simulink library "Vessel"  (R2023a)
settings: Solver=VariableStepAuto  StartTime=0.0  StopTime=10.0  RelTol=1e-3
undefined symbols (not defined in the file): A_ann_aor, alpha1, alpha2, atrium_ventricle, BSA, control, conversion_factor, DAP, DLVP, DP_close_aor, DP_open_aor, DPP, DRVP, E0, E_max, E_min, E_sa_0, E_sv_0, eta, g, K_vc_aor, K_vo_aor, l, L0, lambda, m1, m2, M_rg_aor, M_st_aor, MAP, MPP, n, P0, p_septum_on_off, p_th_on_off, phi, PVR, Q_max, rho, SAP, SI, sigma, SLVP, SPP, SRVP, SVR, t_delay, Ts, UVV_0, V0, V_0, V_max, V_tot, Y_aorta, Y_control
libraries: $bdroot x100, simulink x39, dspsigops x20, slpidlib x11, eeGeneralControl x2, dspstat3 x1
(part 4 of 4)

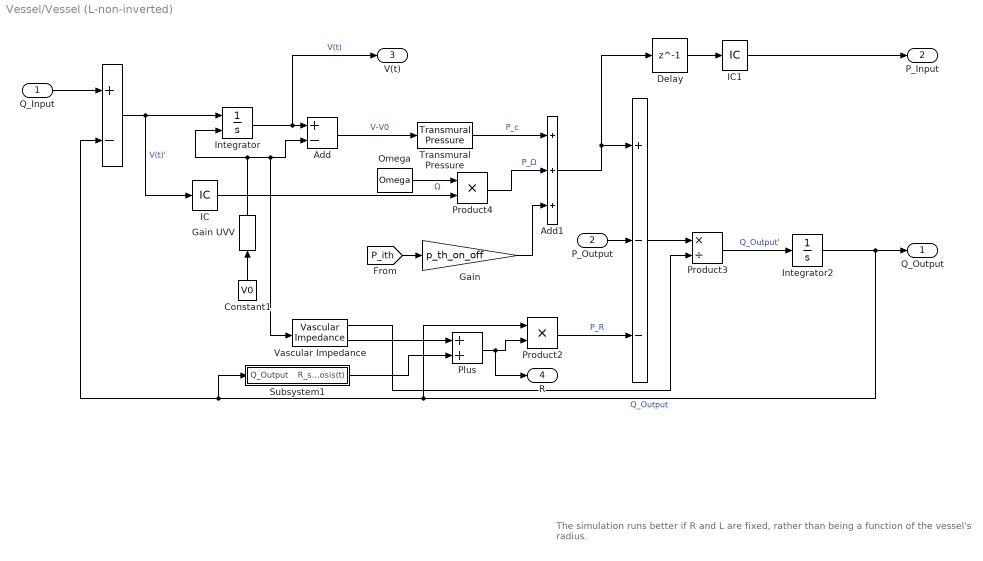
== system Vessel/Vessel (L-non-inverted)  ==
  note: The simulation runs better if R and L are fixed, rather than being a function of the vessel's radius.
  Q_Input : Inport
  P_Output : Inport  Port=2  Unit=mmHg
  " " : Sum  Inputs=+--
  "   " : Sum  Inputs=+-
  Add : Sum  Inputs=+-
  Add1 : Sum  Inputs=+++
  Constant1 : Constant  Value=V0
  Delay : Delay  DelayLength=1  InitialCondition=P0
  Gain : Gain  Gain=p_th_on_off
  Gain UVV : $bdroot/Gain UVV  SystemSampleTime=-1  VariantActivationTime=update diagram  Latency=0  AutoFrameSizeCalculation=off
  IC : InitialCondition  Value=0
  IC1 : InitialCondition  Value=P0
  Integrator : Integrator  InitialConditionSource=external  LimitOutput=on  LowerSaturationLimit=0  ContinuousStateAttributes='Volume'
  Integrator2 : Integrator  LimitOutput=on  UpperSaturationLimit=4000  LowerSaturationLimit=-4000  ContinuousStateAttributes='Flow'
  Omega : $bdroot/Omega  SystemSampleTime=-1  VariantActivationTime=update diagram  Latency=0  AutoFrameSizeCalculation=off
  Plus : Sum
  Product2 : Product
  Product3 : Product  Inputs=*/
  Product4 : Product
  Subsystem1 : Subsystem
  Transmural Pressure : $bdroot/Transmural Pressure  SystemSampleTime=-1  VariantActivationTime=update diagram  Latency=0  AutoFrameSizeCalculation=off
  Vascular Impedance : $bdroot/Vascular Impedance  SystemSampleTime=-1  VariantActivationTime=update diagram  Latency=0  AutoFrameSizeCalculation=off
  Q_Output : Outport
  P_Input : Outport  Port=2
  V(t) : Outport  Port=3
  R : Outport  Port=4
  wires:
  Constant1/1 -> Gain UVV/1
  Integrator2/1 -> Q_Output/1, Product2/1, Subsystem1/1(Q_Output), "   "/2  "Q_Output"
  P_Output/1 -> " "/2
  Omega/1 -> Product4/1  "Ω"
  Product4/1 -> Add1/2  "P_Ω"
  Q_Input/1 -> "   "/1
  Transmural Pressure/1 -> Add1/1  "P_c"
  Add1/1 -> Delay/1, " "/1
  " "/1 -> Product3/1
  Product2/1 -> " "/3  "P_R"
  Add/1 -> Transmural Pressure/1  "V-V0"
  Integrator/1 -> V(t)/1, Add/1  "V(t)"
  "   "/1 -> IC/1, Integrator/1  "V(t)'"
  Product3/1 -> Integrator2/1  "Q_Output'"
  Vascular Impedance/1 -> Product3/2
  [P_ith] -> Gain/1
  Gain/1 -> Add1/3
  IC/1 -> Product4/2
  IC1/1 -> P_Input/1
  Delay/1 -> IC1/1
  Vascular Impedance/2 -> Plus/1
  Plus/1 -> R/1, Product2/2
  Subsystem1/1(R_stenosis(t)) -> Plus/2
  Gain UVV/1 -> Integrator/2, Vascular Impedance/1, Add/2

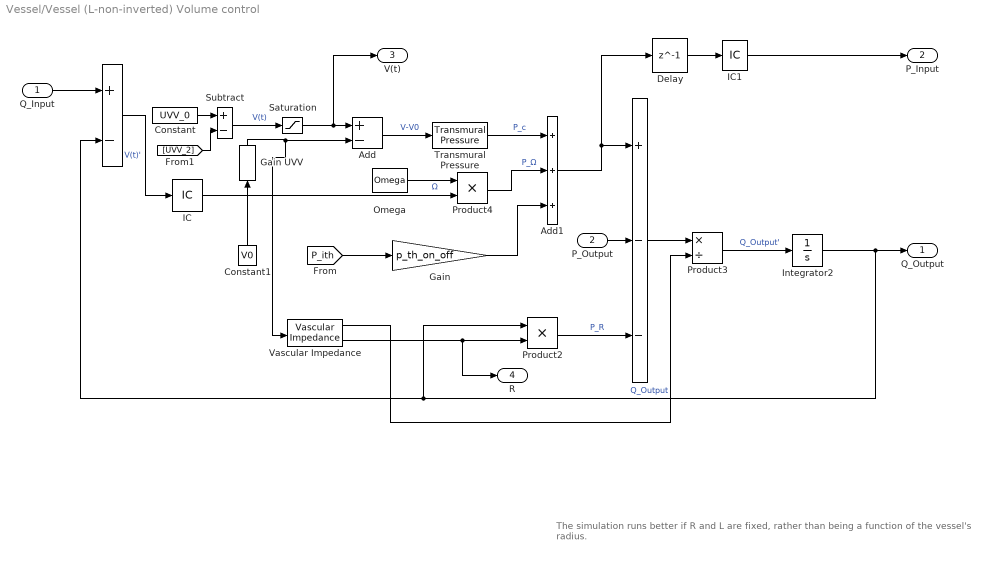
== system Vessel/Vessel (L-non-inverted) Volume control ==
  note: The simulation runs better if R and L are fixed, rather than being a function of the vessel's radius.
  Q_Input : Inport
  P_Output : Inport  Port=2  Unit=mmHg
  " " : Sum  Inputs=+--
  "   " : Sum  Inputs=+-
  Add : Sum  Inputs=+-
  Add1 : Sum  Inputs=+++
  Constant : Constant  Value=UVV_0
  Constant1 : Constant  Value=V0
  Delay : Delay  DelayLength=1  InitialCondition=P0
  Gain : Gain  Gain=p_th_on_off
  Gain UVV : $bdroot/Gain UVV  SystemSampleTime=-1  VariantActivationTime=update diagram  Latency=0  AutoFrameSizeCalculation=off
  IC : InitialCondition  Value=0
  IC1 : InitialCondition  Value=P0
  Integrator2 : Integrator  LimitOutput=on  UpperSaturationLimit=4000  LowerSaturationLimit=-4000  ContinuousStateAttributes='Flow'
  Omega : $bdroot/Omega  SystemSampleTime=-1  VariantActivationTime=update diagram  Latency=0  AutoFrameSizeCalculation=off
  Product2 : Product
  Product3 : Product  Inputs=*/
  Product4 : Product
  Saturation : Saturate  UpperLimit=inf  LowerLimit=0
  Subtract : Sum  Inputs=+-
  Transmural Pressure : $bdroot/Transmural Pressure  SystemSampleTime=-1  VariantActivationTime=update diagram  Latency=0  AutoFrameSizeCalculation=off
  Vascular Impedance : $bdroot/Vascular Impedance  SystemSampleTime=-1  VariantActivationTime=update diagram  Latency=0  AutoFrameSizeCalculation=off
  Q_Output : Outport
  P_Input : Outport  Port=2
  V(t) : Outport  Port=3
  R : Outport  Port=4
  wires:
  Delay/1 -> IC1/1
  IC1/1 -> P_Input/1
  Gain/1 -> Add1/3
  [P_ith] -> Gain/1
  Vascular Impedance/1 -> Product3/2
  Vascular Impedance/2 -> R/1, Product2/2
  Product3/1 -> Integrator2/1  "Q_Output'"
  "   "/1 -> IC/1  "V(t)'"
  Subtract/1 -> Saturation/1  "V(t)"
  Add/1 -> Transmural Pressure/1  "V-V0"
  Product2/1 -> " "/3  "P_R"
  " "/1 -> Product3/1
  Add1/1 -> " "/1, Delay/1
  Transmural Pressure/1 -> Add1/1  "P_c"
  Q_Input/1 -> "   "/1
  Product4/1 -> Add1/2  "P_Ω"
  Omega/1 -> Product4/1  "Ω"
  P_Output/1 -> " "/2
  Integrator2/1 -> "   "/2, Product2/1, Q_Output/1  "Q_Output"
  Constant1/1 -> Gain UVV/1
  [UVV_2] -> Subtract/2
  Constant/1 -> Subtract/1
  Saturation/1 -> Add/1, V(t)/1
  IC/1 -> Product4/2
  Gain UVV/1 -> Vascular Impedance/1, Add/2

== system Vessel/Volume Control ==
  note: OLD
  V_tot(t) : Inport
  Add : Sum  Commented=on
  Constant : Constant  Value=V_tot_0
  Filtered Derivative (Discrete or Continuous) : eeGeneralControl/Filtered Derivative (Discrete or Continuous)  Commented=on  K=1  T=Ts  B=inf  A=-inf  minRatio=1  init_option=Inherited from block input  x0=0  Ts=-1
      settings: LibrarySourceBlock=|
      | ee_sl_lib/General Control/Filtered Derivative
      | (Discrete or Continuous)
  Moving Average : dspstat3/Moving Average  Commented=on  Method=Sliding window  ForgettingFactorPort=off  SpecifyWindowLength=on  WindowLength=4  OverlapLength=3  AllowArbitraryInputLength=off  ForgettingFactor=0.9  SimulateUsing=Code generation
  Subtract : Sum  Inputs=+-
  Switch1 : Switch  Criteria=u2 > Threshold  SaturateOnIntegerOverflow=off  InputSameDT=off
  Q_output : Outport
  wires:
  [V_tot] -> Subtract/2
  Switch1/1 -> Subtract/1
  Subtract/1 -> Q_output/1  "V(t)"
  Filtered Derivative (Discrete or Continuous)/1 -> Add/1
  Constant/1 -> Switch1/3
  V_tot(t)/1 -> Switch1/2, Switch1/1
  Moving Average/1 -> Add/2

== system Vessel/Baroflex control (Fresiello)/Afferent sympathetic activity ==
  P(t) : Inport
  Constant1 : Constant  Value=A*WL
  Constant2 : Constant
  Constant3 : Constant  Value=Paa_SET0
  Constant4 : Constant  Value=Fas_min
  Divide : Product  Inputs=*/
  Gain : Gain  Gain=1/ka
  Gain1 : Gain  Gain=Fas_max
  Math Function : Math
  Minus : Sum  Inputs=-+
  Minus1 : Sum
  Minus2 : Sum
  Minus3 : Sum
  Fas(t) : Outport
  wires:
  Minus1/1 -> Divide/1
  Divide/1 -> Fas(t)/1
  Constant2/1 -> Minus2/2
  Constant4/1 -> Minus1/2
  Gain/1 -> Math Function/1
  P(t)/1 -> Minus/2
  Constant3/1 -> Minus3/2
  Minus/1 -> Gain/1
  Math Function/1 -> Gain1/1, Minus2/1
  Gain1/1 -> Minus1/1
  Minus2/1 -> Divide/2
  Constant1/1 -> Minus3/1
  Minus3/1 -> Minus/1  "Paa_SET"

== system Vessel/Baroflex control (Fresiello)/Efferent sympathetic nerve activity ==
  Fas(t) : Inport
  Constant1 : Constant  Value=B*WL
  Constant4 : Constant  Value=Fes_inf
  Gain : Gain  Gain=-kes
  Gain1 : Gain  Gain=Fes_0-Fes_inf
  Math Function : Math
  Minus2 : Sum  Inputs=+++
  " Fes(t)" : Outport
  wires:
  Math Function/1 -> Gain1/1
  Gain/1 -> Math Function/1
  Fas(t)/1 -> Gain/1
  Gain1/1 -> Minus2/1
  Constant4/1 -> Minus2/2
  Constant1/1 -> Minus2/3  "Δ_Fes"
  Minus2/1 -> " Fes(t)"/1

== system Vessel/Baroflex control (Fresiello)/Efferent vagal nerve activity ==
  Fas(t) : Inport
  " " : Product  Inputs=**
  Constant : Constant
  Constant1 : Constant  Value=C*WL
  Constant2 : Constant  Value=Fas_0
  Constant3 : Constant  Value=Fev_inf0+D*WL
  Constant4 : Constant  Value=Fev_0
  Divide : Product  Inputs=*/
  Gain : Gain  Gain=1/kev
  Math Function : Math
  Minus1 : Sum  Inputs=+-
  Minus2 : Sum
  Minus3 : Sum
  Minus4 : Sum
  " Fev(t)" : Outport
  wires:
  Minus2/1 -> Divide/1
  Constant1/1 -> Minus4/2  "Δ_Fev"
  Constant4/1 -> Minus2/2
  " "/1 -> Minus2/1
  Fas(t)/1 -> Minus1/1
  Gain/1 -> Math Function/1
  Math Function/1 -> Minus3/1, " "/2
  Constant2/1 -> Minus1/2
  Minus1/1 -> Gain/1
  Minus3/1 -> Divide/2
  Constant/1 -> Minus3/2
  Divide/1 -> Minus4/1
  Minus4/1 -> " Fev(t)"/1
  Constant3/1 -> " "/1  "Fev_inf"

== system Vessel/Baroflex control (Fresiello)/Pressure derivation ==
  Paa(t) : Inport
  Filtered Derivative : eeGeneralControl/Filtered Derivative (Discrete or Continuous)  K=1  T=inf  B=inf  A=-inf  minRatio=10  init_option=Inherited from block input  x0=0  Ts=-1
  Gain : Gain  Gain=tau_z
  Gain2 : Gain  Gain=1/tau_p
  Integrator : Integrator
  Minus2 : Sum  Inputs=++-
  P(t) : Outport
  wires:
  Integrator/1 -> Minus2/3, P(t)/1  "P(t)"
  Gain2/1 -> Integrator/1  "P(t)'"
  Paa(t)/1 -> Minus2/2, Filtered Derivative/1  "Paa(t)"
  Filtered Derivative/1 -> Gain/1  "Paa(t)'"
  Gain/1 -> Minus2/1
  Minus2/1 -> Gain2/1

== system Vessel/Baroflex control (Fresiello)/Static sympathetic function ==
  Fes(t) : Inport
  Constant1 : Constant  Value=1.65
  Constant2 : Constant  Value=1.1
  Constant3 : Constant  Value=0
  Gain : Gain  Gain=C_Hs
  Math Function : Math  Operator=log
  Minus : Sum  Inputs=--+
  Minus1 : Sum  Inputs=-+
  Subsystem : Subsystem
  Switch : Switch  Criteria=u2 > Threshold  SaturateOnIntegerOverflow=off  InputSameDT=off
  Transport Delay : TransportDelay  DelayTime=D_Hs
  sf_Hs(t) : Outport
  wires:
  Fes(t)/1 -> Transport Delay/1
  Transport Delay/1 -> Minus/3
  Constant1/1 -> Minus/2
  Constant2/1 -> Minus1/1
  Gain/1 -> sf_Hs(t)/1
  Minus1/1 -> Gain/1
  Subsystem/1(" Fes_SET") -> Minus/1
  Minus/1 -> Math Function/1, Switch/2
  Math Function/1 -> Switch/1
  Switch/1 -> Minus1/2
  Constant3/1 -> Switch/3

== system Vessel/Baroflex control (Fresiello)/Static vagal function ==
  Fev(t) : Inport
  Gain : Gain  Gain=C_Hv
  Minus : Sum  Inputs=-+
  Subsystem : Subsystem
  Transport Delay : TransportDelay  DelayTime=D_Hv
  sf_Hv(t) : Outport
  wires:
  Fev(t)/1 -> Transport Delay/1
  Minus/1 -> Gain/1
  Gain/1 -> sf_Hv(t)/1
  Transport Delay/1 -> Minus/2
  Subsystem/1(" Fev_SET") -> Minus/1

== system Vessel/Carotid Artery (L-non-inverted)/Subsystem1 ==
  Q_Output : Inport
  Abs : Abs  SaturateOnIntegerOverflow=off
  Gain1 : Gain  Gain=SI
  R_stenosis(t) : Outport
  wires:
  Abs/1 -> Gain1/1
  Gain1/1 -> R_stenosis(t)/1
  Q_Output/1 -> Abs/1

== system Vessel/Coarctation (L-non-inverted)/Subsystem ==
  Q_Output : Inport
  Abs : Abs  SaturateOnIntegerOverflow=off
  Gain1 : Gain  Gain=SI*0.000750062
  R_stenosis(t) : Outport
  wires:
  Q_Output/1 -> Abs/1
  Gain1/1 -> R_stenosis(t)/1
  Abs/1 -> Gain1/1

== system Vessel/Heart Chamber1/Pericardial pressure ==
  Vpc : Inport
  Add : Sum
  Add1 : Sum  Inputs=+-+
  Constant : Constant  Value=V_pe
  Constant14 : Constant  Value=P_pc_0
  Constant15 : Constant  Value=V_pc_0
  Constant16 : Constant  Value=phi_pc
  Exp : Math
  Gain : Gain  Gain=K_pc
  Product3 : Product  Inputs=*/
  P_pc : Outport
  wires:
  Add/1 -> P_pc/1
  Exp/1 -> Gain/1
  Constant/1 -> Add1/3
  Constant14/1 -> Add/1
  Vpc/1 -> Add1/1
  Add1/1 -> Product3/1
  Constant15/1 -> Add1/2
  Gain/1 -> Add/2
  Product3/1 -> Exp/1
  Constant16/1 -> Product3/2

== system Vessel/Intrathoracic Pressure/Breathing cycle ==
  Clock : Clock
  Constant : Constant  Value=t_exp+t_ins
  Mod : Math  Operator=mod
  tag scope: t_breathing=global
  wires:
  Mod/1 -> [t_breathing]
  Constant/1 -> Mod/2
  Clock/1 -> Mod/1

== system Vessel/Omega/Subsystem ==
  V-V0 : Inport
  Constant10 : Constant  Value=E0
  Constant11 : Constant  Value=phi
  Math Function1 : Math
  Product1 : Product  Inputs=*/
  Product10 : Product
  E(t) : Outport
  wires:
  Constant11/1 -> Product1/2
  Math Function1/1 -> Product10/1
  Constant10/1 -> Product10/2
  Product10/1 -> E(t)/1  "E(t)"
  Product1/1 -> Math Function1/1
  V-V0/1 -> Product1/1

== system Vessel/SVR Control/Subsystem1 ==
  In1 : Inport
  IsInf : RelationalOperator  Operator=isInf  OutDataTypeStr=boolean  RndMeth=Simplest  InputSameDT=off
  IsNaN : RelationalOperator  Operator=isNaN  OutDataTypeStr=boolean  RndMeth=Simplest  InputSameDT=off
  OR1 : Logic  Operator=OR  IconShape=distinctive  AllPortsSameDT=off  OutDataTypeStr=boolean
  Out1 : Outport
  wires:
  OR1/1 -> Out1/1
  IsNaN/1 -> OR1/2
  IsInf/1 -> OR1/1
  In1/1 -> IsInf/1, IsNaN/1

== system Vessel/SVR Control/Subsystem2 ==
  Signal : Inport
  Trigger : Inport  Port=2
  Memory : Memory
  Switch2 : Switch  Criteria=u2 > Threshold  SaturateOnIntegerOverflow=off  InputSameDT=off
  Out : Outport
  wires:
  Switch2/1 -> Memory/1
  Trigger/1 -> Switch2/2
  Memory/1 -> Out/1, Switch2/3
  Signal/1 -> Switch2/1

== system Vessel/Time varying elastance1/Subsystem ==
  t : Inport
  Data Store Read : DataStoreRead  DataStoreName=T  IndexOptions=Index vector (dialog)  Indices=1  OutputSizes=1
  IsPositive : simulink/Logic and Bit Operations/Compare To Zero  relop=>  OutDataTypeStr=boolean
  Product : Product
  Subsystem : Subsystem
  Subsystem1 : Subsystem
  Subsystem2 : Subsystem
  Subsystem3 : Subsystem
      settings: PortSchema="{\"entries\":[{\"content\":{\"sides\":[{\"content\":{\"connectorIds\":[\"In1\"]},\"type\":\"ConnectorPlacement.EquallySpacedRectSide\",\"uuid\":\"53415d9d-c969-4b15-a3ee-9923cdb17cac\"},{\"content\":{\"connectorIds\":[\"Out1\"],\"side\":\"RIGHT\"},\"type\":\"ConnectorPlacement.EquallySpacedRectSide\",\"uuid\":\"10eb54d7-3431-475c-95dc-df779395c849\"},{\"content\":{\"connectorIds\":[\"In2\",\"In3\"],\"side\":\"TOP\"},\"type\":\"ConnectorPlacement.EquallySpacedRectSide\",\"uuid\":\"aeca1e05-caa4-4591-bcc6-67e67c29b559\"},{\"content\":{\"connectorIds\":[\"In4\",\"In5\"],\"side\":\"BOTTOM\"},\"type\":\"ConnectorPlacement.EquallySpacedRectSide\",\"uuid\":\"6ed2dc98-ea1e-4568-91af-6ae832fd636b\"}]},\"type\":\"ConnectorPlacement.EquallySpacedConnector\",\"uuid\":\"bdfc5c5d-3ff1-4373-b1a6-ef4dafa40c01\"}],\"packageUris\":[\"http://schema.mathworks.com/mf0/Connector/R2020b\"],\"version\":\"1.0\"}"
  Subsystem4 : Subsystem
      settings: PortSchema="{\"entries\":[{\"content\":{\"sides\":[{\"content\":{\"connectorIds\":[\"In1\"]},\"type\":\"ConnectorPlacement.EquallySpacedRectSide\",\"uuid\":\"53415d9d-c969-4b15-a3ee-9923cdb17cac\"},{\"content\":{\"connectorIds\":[\"Out1\"],\"side\":\"RIGHT\"},\"type\":\"ConnectorPlacement.EquallySpacedRectSide\",\"uuid\":\"10eb54d7-3431-475c-95dc-df779395c849\"},{\"content\":{\"connectorIds\":[\"In2\",\"In3\",\"In4\",\"In5\"],\"side\":\"TOP\"},\"type\":\"ConnectorPlacement.EquallySpacedRectSide\",\"uuid\":\"aeca1e05-caa4-4591-bcc6-67e67c29b559\"},{\"content\":{\"connectorIds\":[],\"side\":\"BOTTOM\"},\"type\":\"ConnectorPlacement.EquallySpacedRectSide\",\"uuid\":\"6ed2dc98-ea1e-4568-91af-6ae832fd636b\"}]},\"type\":\"ConnectorPlacement.EquallySpacedConnector\",\"uuid\":\"bdfc5c5d-3ff1-4373-b1a6-ef4dafa40c01\"}],\"packageUris\":[\"http://schema.mathworks.com/mf0/Connector/R2020b\"],\"version\":\"1.0\"}"
  Subtract : Sum  Inputs=+-
  "f(g1, g2)" : Outport
  "f(g1, g2, t-t_delay)" : Outport  Port=2
  wires:
  Product/1 -> Subsystem4/1(t)
  IsPositive/1 -> Product/2
  Subsystem4/1("f(g1, g2, t-t_delay)") -> "f(g1, g2, t-t_delay)"/1
  Subtract/1 -> Product/1, IsPositive/1
  Subsystem2/1(t_delay) -> Subtract/2
  Subsystem3/1("f(g1, g2)") -> "f(g1, g2)"/1
  Subsystem1/2(tau2) -> Subsystem3/5(tau2), Subsystem4/2(tau2)
  t/1 -> Subsystem3/1(t), Subtract/1
  Subsystem1/1(tau1) -> Subsystem3/4(tau1), Subsystem4/3(tau1)
  Subsystem/2(m2) -> Subsystem4/4(m2), Subsystem3/2(m2)
  Subsystem/1(m1) -> Subsystem4/5(m1), Subsystem3/3(m1)
  Data Store Read/1 -> Subsystem/1(T), Subsystem1/1(T), Subsystem2/1(T)

== system Vessel/Time varying elastance1/e_max ==
  v_ed : Inport
  V' : Inport  Port=2
  " " : Constant  Value=E_max
  Bias : Bias  Bias=1  SaturateOnIntegerOverflow=off
  Bias1 : Bias  Bias=1  SaturateOnIntegerOverflow=off
  Constant12 : Constant  Value=Q_max
  Constant3 : Constant  Value=4
  Constant9 : Constant  Value=V_max
  Divide3 : Product  Inputs=*/
  Divide4 : Product  Inputs=***
  Divide5 : Product  Inputs=*/
  Gain : Gain  Gain=-1
  Gain1 : Gain  Gain=-1
  Gain_E_max : $bdroot/Gain_E_max  SystemSampleTime=-1  VariantActivationTime=update diagram  Latency=0  AutoFrameSizeCalculation=off
  Power1 : Math  Operator=pow
  e_max : Outport
  wires:
  Power1/1 -> Gain/1
  Gain1/1 -> Bias1/1
  Constant9/1 -> Divide5/2
  Divide5/1 -> Power1/1
  Gain/1 -> Bias/1
  Bias/1 -> Divide4/1
  Bias1/1 -> Divide4/3
  v_ed/1 -> Divide5/1
  Constant3/1 -> Power1/2
  Constant12/1 -> Divide3/2
  V'/1 -> Divide3/1
  Divide3/1 -> Gain1/1
  " "/1 -> Gain_E_max/1
  Gain_E_max/1 -> Divide4/2
  Divide4/1 -> e_max/1  "e_max"

== system Vessel/Time varying elastance1/e_min ==
  V : Inport
  Constant5 : Constant  Value=E_min
  Constant6 : Constant  Value=sigma
  Constant8 : Constant  Value=V_0
  Exp : Math
  Gain_E_min : $bdroot/Gain_E_min  SystemSampleTime=-1  VariantActivationTime=update diagram  Latency=0  AutoFrameSizeCalculation=off
  Product1 : Product
  Product2 : Product
  Subtract : Sum  Inputs=+-
  e_min : Outport
  wires:
  Constant6/1 -> Product2/1
  Constant5/1 -> Gain_E_min/1
  V/1 -> Subtract/1
  Exp/1 -> Product1/1
  Product2/1 -> Exp/1  "m1"
  Subtract/1 -> Product2/2
  Product1/1 -> e_min/1  "e_min"
  Constant8/1 -> Subtract/2
  Gain_E_min/1 -> Product1/2

== system Vessel/Time varying elastance1/k ==
  t : Inport
  "f(g1, g2)" : Inport  Port=2
  e_max : Inport  Port=3
  e_min : Inport  Port=4
  Divide : Product  Inputs=/*
  Subsystem1 : Subsystem
  Subtract : Sum  Inputs=+-
  k : Outport
  wires:
  Divide/1 -> k/1  "k"
  Subtract/1 -> Divide/2
  e_min/1 -> ?
  "f(g1, g2)"/1 -> Subsystem1/2("f(g1, g2)")
  t/1 -> Subsystem1/1(t)
  Subsystem1/1("max(f(g1, g2))") -> Divide/1
  e_max/1 -> Subtract/1

== system Vessel/Total heart/Aortic Flow Target ==
  Q_aorta_target : Inport
  "Q_aorta " : Inport  Port=2
  Subsystem : Subsystem
  Switch1 : Switch  Criteria=u2 ~= 0  SaturateOnIntegerOverflow=off  InputSameDT=off
  Q_aorta : Outport
  wires:
  Q_aorta_target/1 -> Subsystem/1(In1), Switch1/1
  Switch1/1 -> Q_aorta/1
  "Q_aorta "/1 -> Switch1/3
  Subsystem/1(Out1) -> Switch1/2

== system Vessel/Total heart/Diastolic Pressur1 ==
  P_in : Inport
  MinMax Running Resettable : simulink/Math Operations/MinMax Running Resettable  Function=min  vinit=300
      settings: AttributesFormatString=%<vinit>
  Pulse Generator1 : DiscretePulseGenerator  PulseType=Time based  TimeSource=Use external signal  Period=100  PulseWidth=1e-3
  Sample and Hold1 : dspsigops/Sample and Hold  trig=Rising edge  initCond=0  latchinput=on
  P_dys : Outport
  wires:
  MinMax Running Resettable/1 -> Sample and Hold1/1
  [t_b] -> Pulse Generator1/1
  P_in/1 -> MinMax Running Resettable/1
  Pulse Generator1/1 -> MinMax Running Resettable/2, Sample and Hold1/Trigger
  Sample and Hold1/1 -> P_dys/1

== system Vessel/Total heart/Diastolic Pressur2 ==
  P_in : Inport
  MinMax Running Resettable : simulink/Math Operations/MinMax Running Resettable  Function=min  vinit=300
      settings: AttributesFormatString=%<vinit>
  Pulse Generator1 : DiscretePulseGenerator  PulseType=Time based  TimeSource=Use external signal  Period=100  PulseWidth=1e-3
  Sample and Hold1 : dspsigops/Sample and Hold  trig=Rising edge  initCond=0  latchinput=on
  P_dys : Outport
  wires:
  Sample and Hold1/1 -> P_dys/1
  Pulse Generator1/1 -> Sample and Hold1/Trigger, MinMax Running Resettable/2
  P_in/1 -> MinMax Running Resettable/1
  [t_b] -> Pulse Generator1/1
  MinMax Running Resettable/1 -> Sample and Hold1/1

== system Vessel/Total heart/Diastolic Pressur3 ==
  P_in : Inport
  MinMax Running Resettable : simulink/Math Operations/MinMax Running Resettable  Function=min  vinit=300
      settings: AttributesFormatString=%<vinit>
  Pulse Generator1 : DiscretePulseGenerator  PulseType=Time based  TimeSource=Use external signal  Period=100  PulseWidth=1e-3
  Sample and Hold1 : dspsigops/Sample and Hold  trig=Rising edge  initCond=0  latchinput=on
  P_dys : Outport
  wires:
  MinMax Running Resettable/1 -> Sample and Hold1/1
  [t_b] -> Pulse Generator1/1
  P_in/1 -> MinMax Running Resettable/1
  Pulse Generator1/1 -> MinMax Running Resettable/2, Sample and Hold1/Trigger
  Sample and Hold1/1 -> P_dys/1

== system Vessel/Total heart/Diastolic Pressur4 ==
  P_in : Inport
  MinMax Running Resettable : simulink/Math Operations/MinMax Running Resettable  Function=min  vinit=300
      settings: AttributesFormatString=%<vinit>
  Pulse Generator1 : DiscretePulseGenerator  PulseType=Time based  TimeSource=Use external signal  Period=100  PulseWidth=1e-3
  Sample and Hold1 : dspsigops/Sample and Hold  trig=Rising edge  initCond=0  latchinput=on
  P_dys : Outport
  wires:
  MinMax Running Resettable/1 -> Sample and Hold1/1
  [t_b] -> Pulse Generator1/1
  P_in/1 -> MinMax Running Resettable/1
  Pulse Generator1/1 -> MinMax Running Resettable/2, Sample and Hold1/Trigger
  Sample and Hold1/1 -> P_dys/1

== system Vessel/Total heart/Diastolic Pressur5 ==
  P_in : Inport
  MinMax Running Resettable : simulink/Math Operations/MinMax Running Resettable  Function=min  vinit=300
      settings: AttributesFormatString=%<vinit>
  Pulse Generator1 : DiscretePulseGenerator  PulseType=Time based  TimeSource=Use external signal  Period=100  PulseWidth=1e-3
  Sample and Hold1 : dspsigops/Sample and Hold  trig=Rising edge  initCond=0  latchinput=on
  P_dys : Outport
  wires:
  Sample and Hold1/1 -> P_dys/1
  Pulse Generator1/1 -> Sample and Hold1/Trigger, MinMax Running Resettable/2
  P_in/1 -> MinMax Running Resettable/1
  [t_b] -> Pulse Generator1/1
  MinMax Running Resettable/1 -> Sample and Hold1/1

== system Vessel/Total heart/Heart beat ==
  note: This algorithm is able to generate a time varying cardiac cylce. use this one if you wnat to implement the baroflex control
  Clock : Clock  Commented=on
  Clock1 : Clock  Commented=on
      settings: Decimation=1000
  Constant2 : Constant
  Counter : $bdroot/Counter  SystemSampleTime=-1  VariantActivationTime=update diagram  Latency=0  AutoFrameSizeCalculation=off
  Data Store Read : DataStoreRead  Commented=on  DataStoreName=T  IndexOptions=Index vector (dialog)  Indices=1  OutputSizes=1
  Data Store Read1 : DataStoreRead  DataStoreName=T  IndexOptions=Index vector (dialog)  Indices=1  OutputSizes=1
  Goto : Goto  Commented=on  GotoTag=t_b  TagVisibility=global
  Memory1 : Memory  InheritSampleTime=on
  Memory2 : Memory  InheritSampleTime=on
  Minus2 : Sum  Inputs=+-
  Minus3 : Sum
  Mod : Math  Commented=on  Operator=mod
  Mod1 : Math  Operator=mod
  Product : Product
  Product1 : Product
  Reciprocal : Product  Inputs=/
  Subsystem : Subsystem  Commented=on
      settings: PortSchema="{\"entries\":[{\"content\":{\"sides\":[{\"content\":{\"connectorIds\":[]},\"type\":\"ConnectorPlacement.EquallySpacedRectSide\",\"uuid\":\"b0d09b2a-d6a3-40e8-ba7a-f77784391b40\"},{\"content\":{\"connectorIds\":[],\"side\":\"RIGHT\"},\"type\":\"ConnectorPlacement.EquallySpacedRectSide\",\"uuid\":\"9ef2e8f0-226d-4f4a-9954-6d467dae8c6d\"},{\"content\":{\"connectorIds\":[],\"side\":\"TOP\"},\"type\":\"ConnectorPlacement.EquallySpacedRectSide\",\"uuid\":\"f2c26a28-50d3-4f37-a9aa-276f629de1b6\"},{\"content\":{\"connectorIds\":[\"In1\"],\"side\":\"BOTTOM\"},\"type\":\"ConnectorPlacement.EquallySpacedRectSide\",\"uuid\":\"81f5763a-3fea-4455-9747-ce77221053da\"}]},\"type\":\"ConnectorPlacement.EquallySpacedConnector\",\"uuid\":\"c94cfed1-1e93-49fe-89a1-fd142b1a38b7\"}],\"packageUris\":[\"http://schema.mathworks.com/mf0/Connector/R2020b\"],\"version\":\"1.0\"}"
  To Workspace : ToWorkspace  VariableName=T  SampleTime=-1
  tag scope: t_b=global
  wires:
  Mod/1 -> Goto/1
  Data Store Read/1 -> Mod/2
  Clock/1 -> Mod/1
  Mod1/1 -> Memory2/1, Product1/1
  Minus2/1 -> Product/1
  Product1/1 -> [t_b]
  Memory2/1 -> Minus3/1
  Memory1/1 -> Minus2/2
  Minus3/1 -> Mod1/1
  Constant2/1 -> Mod1/2
  Product/1 -> Minus3/2
  Data Store Read1/1 -> Reciprocal/1, To Workspace/1, Product1/2  "T"
  Reciprocal/1 -> Product/2
  Counter/1 -> Minus2/1, Subsystem/1(t), Memory1/1

== system Vessel/Total heart/Left Atrial Pressure Target ==
  P_LA_target : Inport
  "P_LA " : Inport  Port=2
  Subsystem : $bdroot/Total heart/Aortic Flow Target/Subsystem  SystemSampleTime=-1  VariantActivationTime=update diagram  Latency=0  AutoFrameSizeCalculation=off
  Switch1 : Switch  Criteria=u2 ~= 0  SaturateOnIntegerOverflow=off  InputSameDT=off
  P_LA : Outport
  wires:
  P_LA_target/1 -> Subsystem/1, Switch1/1
  Switch1/1 -> P_LA/1
  "P_LA "/1 -> Switch1/3
  Subsystem/1 -> Switch1/2

== system Vessel/Total heart/MAP1 ==
  P_ao : Inport
  Data Store Read1 : DataStoreRead  DataStoreName=T  IndexOptions=Index vector (dialog)  Indices=1  OutputSizes=1
  Divide : Product  Inputs=/*
  Integrator : Integrator  ExternalReset=falling
  Pulse Generator : DiscretePulseGenerator  PulseType=Time based  TimeSource=Use external signal  Period=100  PulseWidth=1e-3
  Sample and Hold : dspsigops/Sample and Hold  trig=Rising edge  initCond=0  latchinput=off
  MAP : Outport
  wires:
  P_ao/1 -> Integrator/1
  Data Store Read1/1 -> Divide/1
  Divide/1 -> MAP/1
  [t_b] -> Pulse Generator/1
  Pulse Generator/1 -> Sample and Hold/Trigger, Integrator/2
  Integrator/1 -> Sample and Hold/1
  Sample and Hold/1 -> Divide/2

== system Vessel/Total heart/MAP2 ==
  P_ao : Inport
  Data Store Read1 : DataStoreRead  DataStoreName=T  IndexOptions=Index vector (dialog)  Indices=1  OutputSizes=1
  Divide : Product  Inputs=/*
  Integrator : Integrator  ExternalReset=falling
  Pulse Generator : DiscretePulseGenerator  PulseType=Time based  TimeSource=Use external signal  Period=100  PulseWidth=1e-3
  Sample and Hold : dspsigops/Sample and Hold  trig=Rising edge  initCond=0  latchinput=off
  MAP : Outport
  wires:
  Sample and Hold/1 -> Divide/2
  Integrator/1 -> Sample and Hold/1
  Pulse Generator/1 -> Integrator/2, Sample and Hold/Trigger
  [t_b] -> Pulse Generator/1
  Divide/1 -> MAP/1
  Data Store Read1/1 -> Divide/1
  P_ao/1 -> Integrator/1

== system Vessel/Total heart/MAP3 ==
  P_ao : Inport
  Data Store Read1 : DataStoreRead  DataStoreName=T  IndexOptions=Index vector (dialog)  Indices=1  OutputSizes=1
  Divide : Product  Inputs=/*
  Integrator : Integrator  ExternalReset=falling
  Pulse Generator : DiscretePulseGenerator  PulseType=Time based  TimeSource=Use external signal  Period=100  PulseWidth=1e-3
  Sample and Hold : dspsigops/Sample and Hold  trig=Rising edge  initCond=0  latchinput=off
  MAP : Outport
  wires:
  P_ao/1 -> Integrator/1
  Data Store Read1/1 -> Divide/1
  Divide/1 -> MAP/1
  [t_b] -> Pulse Generator/1
  Pulse Generator/1 -> Sample and Hold/Trigger, Integrator/2
  Integrator/1 -> Sample and Hold/1
  Sample and Hold/1 -> Divide/2

== system Vessel/Total heart/Pericardial Volume ==
  Add2 : Sum  Inputs=++++
  To Workspace : ToWorkspace  VariableName=V_RA  SampleTime=-1
  To Workspace1 : ToWorkspace  VariableName=V_LV  SampleTime=-1
  To Workspace2 : ToWorkspace  VariableName=V_RV  SampleTime=-1
  To Workspace3 : ToWorkspace  VariableName=V_LA  SampleTime=-1
  tag scope: V_pc=global
  wires:
  [V_LV] -> To Workspace1/1, Add2/4
  [V_RA] -> To Workspace/1, Add2/1
  [V_LA] -> To Workspace3/1, Add2/3
  Add2/1 -> [V_pc]
  [V_RV] -> To Workspace2/1, Add2/2

== system Vessel/Total heart/Pulmonary Flow ==
  Q_pulmonary_target : Inport
  "Q_pulmonary " : Inport  Port=2
  Subsystem : $bdroot/Total heart/Aortic Flow Target/Subsystem  SystemSampleTime=-1  VariantActivationTime=update diagram  Latency=0  AutoFrameSizeCalculation=off
  Switch1 : Switch  Criteria=u2 ~= 0  SaturateOnIntegerOverflow=off  InputSameDT=off
  Q_pulmonary : Outport
  wires:
  "Q_pulmonary "/1 -> Switch1/3
  Switch1/1 -> Q_pulmonary/1
  Q_pulmonary_target/1 -> Switch1/1, Subsystem/1
  Subsystem/1 -> Switch1/2

== system Vessel/Total heart/Right Atrial Pressure Target ==
  P_RA_target : Inport
  "P_RA " : Inport  Port=2
  Subsystem : $bdroot/Total heart/Aortic Flow Target/Subsystem  SystemSampleTime=-1  VariantActivationTime=update diagram  Latency=0  AutoFrameSizeCalculation=off
  Switch1 : Switch  Criteria=u2 ~= 0  SaturateOnIntegerOverflow=off  InputSameDT=off
  P_RA : Outport
  wires:
  "P_RA "/1 -> Switch1/3
  Switch1/1 -> P_RA/1
  P_RA_target/1 -> Switch1/1, Subsystem/1
  Subsystem/1 -> Switch1/2

== system Vessel/Total heart/Systolic Pressure1 ==
  P_in : Inport
  MinMax Running Resettable1 : simulink/Math Operations/MinMax Running Resettable  Function=max  vinit=0
      settings: AttributesFormatString=%<vinit>
  Pulse Generator1 : DiscretePulseGenerator  PulseType=Time based  TimeSource=Use external signal  Period=100  PulseWidth=1e-3
  Sample and Hold1 : dspsigops/Sample and Hold  trig=Rising edge  initCond=0  latchinput=on
  P_sys : Outport
  wires:
  MinMax Running Resettable1/1 -> Sample and Hold1/1
  Pulse Generator1/1 -> MinMax Running Resettable1/2, Sample and Hold1/Trigger
  Sample and Hold1/1 -> P_sys/1
  P_in/1 -> MinMax Running Resettable1/1
  [t_b] -> Pulse Generator1/1

== system Vessel/Total heart/Systolic Pressure2 ==
  P_in : Inport
  MinMax Running Resettable1 : simulink/Math Operations/MinMax Running Resettable  Function=max  vinit=0
      settings: AttributesFormatString=%<vinit>
  Pulse Generator1 : DiscretePulseGenerator  PulseType=Time based  TimeSource=Use external signal  Period=100  PulseWidth=1e-3
  Sample and Hold1 : dspsigops/Sample and Hold  trig=Rising edge  initCond=0  latchinput=on
  P_sys : Outport
  wires:
  [t_b] -> Pulse Generator1/1
  P_in/1 -> MinMax Running Resettable1/1
  Sample and Hold1/1 -> P_sys/1
  Pulse Generator1/1 -> Sample and Hold1/Trigger, MinMax Running Resettable1/2
  MinMax Running Resettable1/1 -> Sample and Hold1/1

== system Vessel/Total heart/Systolic Pressure3 ==
  P_in : Inport
  MinMax Running Resettable1 : simulink/Math Operations/MinMax Running Resettable  Function=max  vinit=0
      settings: AttributesFormatString=%<vinit>
  Pulse Generator1 : DiscretePulseGenerator  PulseType=Time based  TimeSource=Use external signal  Period=100  PulseWidth=1e-3
  Sample and Hold1 : dspsigops/Sample and Hold  trig=Rising edge  initCond=0  latchinput=on
  P_sys : Outport
  wires:
  MinMax Running Resettable1/1 -> Sample and Hold1/1
  Pulse Generator1/1 -> MinMax Running Resettable1/2, Sample and Hold1/Trigger
  Sample and Hold1/1 -> P_sys/1
  P_in/1 -> MinMax Running Resettable1/1
  [t_b] -> Pulse Generator1/1

== system Vessel/Total heart/Systolic Pressure4 ==
  P_in : Inport
  MinMax Running Resettable1 : simulink/Math Operations/MinMax Running Resettable  Function=max  vinit=0
      settings: AttributesFormatString=%<vinit>
  Pulse Generator1 : DiscretePulseGenerator  PulseType=Time based  TimeSource=Use external signal  Period=100  PulseWidth=1e-3
  Sample and Hold1 : dspsigops/Sample and Hold  trig=Rising edge  initCond=0  latchinput=on
  P_sys : Outport
  wires:
  MinMax Running Resettable1/1 -> Sample and Hold1/1
  Pulse Generator1/1 -> MinMax Running Resettable1/2, Sample and Hold1/Trigger
  Sample and Hold1/1 -> P_sys/1
  P_in/1 -> MinMax Running Resettable1/1
  [t_b] -> Pulse Generator1/1

== system Vessel/Total heart/Systolic Pressure5 ==
  P_in : Inport
  MinMax Running Resettable1 : simulink/Math Operations/MinMax Running Resettable  Function=max  vinit=0
      settings: AttributesFormatString=%<vinit>
  Pulse Generator1 : DiscretePulseGenerator  PulseType=Time based  TimeSource=Use external signal  Period=100  PulseWidth=1e-3
  Sample and Hold1 : dspsigops/Sample and Hold  trig=Rising edge  initCond=0  latchinput=on
  P_sys : Outport
  wires:
  [t_b] -> Pulse Generator1/1
  P_in/1 -> MinMax Running Resettable1/1
  Sample and Hold1/1 -> P_sys/1
  Pulse Generator1/1 -> Sample and Hold1/Trigger, MinMax Running Resettable1/2
  MinMax Running Resettable1/1 -> Sample and Hold1/1

== system Vessel/Transeptal pressure/Subsystem ==
  Add1 : Sum  Inputs=+-
  Constant : Constant  Value=atrium_ventricle
  Constant1 : Constant
  Out1 : Outport
  wires:
  Add1/1 -> Out1/1
  Constant1/1 -> Add1/2
  Constant/1 -> Add1/1

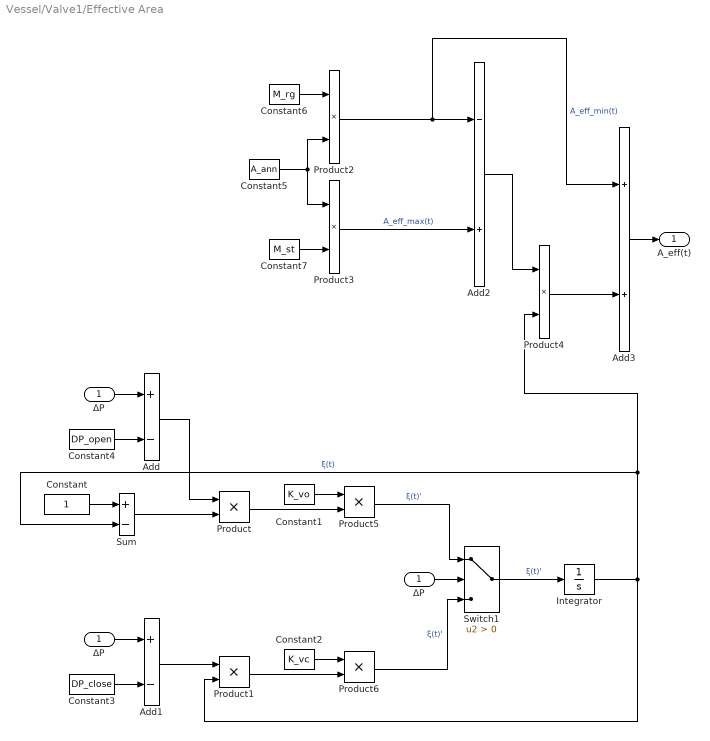
== system Vessel/Valve1/Effective Area ==
  "ΔP  " : Inport
  Add : Sum  Inputs=+-
  Add1 : Sum  Inputs=+-
  Add2 : Sum  Inputs=-+
  Add3 : Sum
  Constant : Constant
  Constant1 : Constant  Value=K_vo
  Constant2 : Constant  Value=K_vc
  Constant3 : Constant  Value=DP_close
  Constant4 : Constant  Value=DP_open
  Constant5 : Constant  Value=A_ann
  Constant6 : Constant  Value=M_rg
  Constant7 : Constant  Value=M_st
  Integrator : Integrator  LimitOutput=on  UpperSaturationLimit=1  LowerSaturationLimit=0
  Product{,1..6} (7 alike) : Product
  Sum : Sum  Inputs=+-
  Switch1 : Switch  Criteria=u2 > Threshold  SaturateOnIntegerOverflow=off  InputSameDT=off
  "ΔP " : InportShadow
  "ΔP     " : InportShadow
  A_eff(t) : Outport
  wires:
  "ΔP     "/1 -> Switch1/2
  Switch1/1 -> Integrator/1  "ξ(t)'"
  Constant7/1 -> Product3/2
  Constant2/1 -> Product6/1
  Constant1/1 -> Product5/1
  Product5/1 -> Switch1/1  "ξ(t)'"
  Constant/1 -> Sum/1
  Constant4/1 -> Add/2
  "ΔP  "/1 -> Add/1
  Sum/1 -> Product/2
  Add/1 -> Product/1
  Product/1 -> Product5/2
  Add1/1 -> Product1/1
  Product1/1 -> Product6/2
  Constant3/1 -> Add1/2
  Product6/1 -> Switch1/3  "ξ(t)'"
  "ΔP "/1 -> Add1/1
  Integrator/1 -> Product4/2, Sum/2, Product1/2  "ξ(t)"
  Constant6/1 -> Product2/1
  Constant5/1 -> Product3/1, Product2/2
  Product2/1 -> Add2/1, Add3/1  "A_eff_min(t)"
  Product3/1 -> Add2/2  "A_eff_max(t)"
  Add2/1 -> Product4/1
  Product4/1 -> Add3/2
  Add3/1 -> A_eff(t)/1

== system Vessel/Valve1/Subsystem ==
  A_eff(t) : Inport
  Gain : Gain  Gain=rho/2/(980.665*1.3595101283313)
  Gain1 : Gain  Gain=rho*2/pi/(980.665*1.3595101283313)
  Reciprocal : Product  Inputs=/
  Reciprocal1 : Product  Inputs=/
  Square : Math  Operator=square
  radius : Subsystem
  B_Valve : Outport
  L_Valve : Outport  Port=2
  wires:
  Gain1/1 -> L_Valve/1  "L_Valve"
  Square/1 -> Reciprocal/1
  A_eff(t)/1 -> Square/1, radius/1(A_eff(t))
  Reciprocal1/1 -> Gain1/1
  radius/1(r(t)) -> Reciprocal1/1
  Gain/1 -> B_Valve/1  "B_Valve"
  Reciprocal/1 -> Gain/1

== system Vessel/Vessel (L-non-inverted) /Subsystem1 ==
  Q_Output : Inport
  Abs : Abs  SaturateOnIntegerOverflow=off
  Gain1 : Gain  Gain=SI
  R_stenosis(t) : Outport
  wires:
  Abs/1 -> Gain1/1
  Gain1/1 -> R_stenosis(t)/1
  Q_Output/1 -> Abs/1

== system Vessel/Baroflex control (Fresiello)/Static sympathetic function/Subsystem ==
  Afferent sympathetic activity : $bdroot/Baroflex control (Fresiello)/Afferent sympathetic  activity  SystemSampleTime=-1  VariantActivationTime=update diagram  Latency=0  AutoFrameSizeCalculation=off
  Constant3 : Constant  Value=A*WL
  Constant4 : Constant  Value=Paa_SET0
  Efferent sympathetic nerve activity : $bdroot/Baroflex control (Fresiello)/Efferent sympathetic  nerve activity  SystemSampleTime=-1  VariantActivationTime=update diagram  Latency=0  AutoFrameSizeCalculation=off
  Minus3 : Sum
  Pressure derivation : $bdroot/Baroflex control (Fresiello)/Pressure derivation  SystemSampleTime=-1  VariantActivationTime=update diagram  Latency=0  AutoFrameSizeCalculation=off
  " Fes_SET" : Outport
  wires:
  Efferent sympathetic nerve activity/1 -> " Fes_SET"/1
  Constant3/1 -> Minus3/1
  Minus3/1 -> Pressure derivation/1  "Paa_SET"
  Pressure derivation/1 -> Afferent sympathetic activity/1
  Constant4/1 -> Minus3/2
  Afferent sympathetic activity/1 -> Efferent sympathetic nerve activity/1

== system Vessel/Baroflex control (Fresiello)/Static vagal function/Subsystem ==
  Afferent sympathetic activity : $bdroot/Baroflex control (Fresiello)/Afferent sympathetic  activity  SystemSampleTime=-1  VariantActivationTime=update diagram  Latency=0  AutoFrameSizeCalculation=off
  Constant1 : Constant  Value=A*WL
  Constant3 : Constant  Value=Paa_SET0
  Efferent vagal nerve activity : $bdroot/Baroflex control (Fresiello)/Efferent vagal  nerve activity  SystemSampleTime=-1  VariantActivationTime=update diagram  Latency=0  AutoFrameSizeCalculation=off
  Minus3 : Sum
  Pressure derivation : $bdroot/Baroflex control (Fresiello)/Pressure derivation  SystemSampleTime=-1  VariantActivationTime=update diagram  Latency=0  AutoFrameSizeCalculation=off
  " Fev_SET" : Outport
  wires:
  Efferent vagal nerve activity/1 -> " Fev_SET"/1
  Minus3/1 -> Pressure derivation/1  "Paa_SET"
  Constant1/1 -> Minus3/1
  Constant3/1 -> Minus3/2
  Pressure derivation/1 -> Afferent sympathetic activity/1
  Afferent sympathetic activity/1 -> Efferent vagal nerve activity/1

== system Vessel/Time varying elastance1/Subsystem/Subsystem ==
  T : Inport
  Constant : Constant  Value=m1
  Constant1 : Constant  Value=m2
  Constant2 : Constant  Value=0.4937
  Constant3 : Constant  Value=-0.5024
  Power : Math  Operator=pow
  Power1 : Math  Operator=pow
  Product : Product
  Product1 : Product
  m1 : Outport
  m2 : Outport  Port=2
  wires:
  Product1/1 -> m2/1  "m2"
  T/1 -> Power1/1, Power/1
  Constant1/1 -> Product1/2
  Product/1 -> m1/1  "m1"
  Constant/1 -> Product/1
  Power/1 -> Product/2
  Power1/1 -> Product1/1
  Constant2/1 -> Power/2
  Constant3/1 -> Power1/2

== system Vessel/Time varying elastance1/Subsystem/Subsystem1 ==
  T : Inport
  Constant1 : Constant  Value=-0.6993
  Constant10 : Constant  Value=alpha2
  Constant2 : Constant  Value=-0.7033
  Constant7 : Constant  Value=alpha1
  Divide1 : Product  Inputs=**
  Divide2 : Product  Inputs=**
  Power1 : Math  Operator=pow
  Power2 : Math  Operator=pow
  Product1 : Product
  Product2 : Product
  T1 : InportShadow
  tau1 : Outport
  tau2 : Outport  Port=2
  wires:
  Product1/1 -> tau1/1  "tau1"
  Constant10/1 -> Divide2/2
  Constant7/1 -> Divide1/1
  Product2/1 -> tau2/1  "tau2"
  Divide2/1 -> Product2/2  "alpha2"
  Divide1/1 -> Product1/1  "alpha1"
  T/1 -> Product2/1, Product1/2
  Constant1/1 -> Power1/2
  Power1/1 -> Divide1/2
  Constant2/1 -> Power2/2
  Power2/1 -> Divide2/1
  T1/1 -> Power1/1, Power2/1

== system Vessel/Time varying elastance1/Subsystem/Subsystem2 ==
  T : Inport
  Constant1 : Constant  Value=0.9958
  Constant2 : Constant  Value=t_delay
  Power1 : Math  Operator=pow
  Product1 : Product
  t_delay : Outport
  wires:
  Product1/1 -> t_delay/1  "t_delay"
  Power1/1 -> Product1/2
  T/1 -> Power1/1
  Constant2/1 -> Product1/1
  Constant1/1 -> Power1/2

== system Vessel/Time varying elastance1/Subsystem/Subsystem3 ==
  t : Inport
  m2 : Inport  Port=2
  m1 : Inport  Port=3
  tau1 : Inport  Port=4
  tau2 : Inport  Port=5
  Bias : Bias  Bias=1  SaturateOnIntegerOverflow=off
  Bias1 : Bias  Bias=1  SaturateOnIntegerOverflow=off
  Divide1 : Product  Inputs=*/
  Divide2 : Product  Inputs=**
  Divide3 : Product  Inputs=/*
  Divide4 : Product  Inputs=*/
  Power1 : Math  Operator=pow
  Power2 : Math  Operator=pow
  Reciprocal : Product  Inputs=/
  "f(g1, g2)" : Outport
  wires:
  tau1/1 -> Divide3/1
  m1/1 -> Power1/2
  Divide2/1 -> "f(g1, g2)"/1  "f(g1, g2)"
  tau2/1 -> Divide4/2
  Reciprocal/1 -> Divide2/2  "1/(1+g2)"
  Bias1/1 -> Reciprocal/1  "1+g2"
  Power2/1 -> Bias1/1  "g2"
  Power1/1 -> Divide1/1, Bias/1  "g1"
  t/1 -> Divide4/1, Divide3/2
  Divide1/1 -> Divide2/1  "g1/(1+g1)"
  Bias/1 -> Divide1/2  "1+g1"
  Divide4/1 -> Power2/1
  m2/1 -> Power2/2
  Divide3/1 -> Power1/1

== system Vessel/Time varying elastance1/Subsystem/Subsystem4 ==
  t : Inport
  tau2 : Inport  Port=2
  tau1 : Inport  Port=3
  m2 : Inport  Port=4
  m1 : Inport  Port=5
  Bias : Bias  Bias=1  SaturateOnIntegerOverflow=off
  Bias1 : Bias  Bias=1  SaturateOnIntegerOverflow=off
  Divide1 : Product  Inputs=*/
  Divide2 : Product  Inputs=**
  Divide3 : Product  Inputs=/*
  Divide4 : Product  Inputs=*/
  Power1 : Math  Operator=pow
  Power2 : Math  Operator=pow
  Reciprocal : Product  Inputs=/
  "f(g1, g2, t-t_delay)" : Outport
  wires:
  Divide3/1 -> Power1/1
  m2/1 -> Power2/2
  Divide4/1 -> Power2/1
  Bias/1 -> Divide1/2  "1+g1"
  Divide1/1 -> Divide2/1  "g1/(1+g1)"
  t/1 -> Divide4/1, Divide3/2
  Power1/1 -> Bias/1, Divide1/1  "g1"
  Power2/1 -> Bias1/1  "g2"
  Bias1/1 -> Reciprocal/1  "1+g2"
  Reciprocal/1 -> Divide2/2  "1/(1+g2)"
  tau2/1 -> Divide4/2
  Divide2/1 -> "f(g1, g2, t-t_delay)"/1  "f(g1, g2)"
  m1/1 -> Power1/2
  tau1/1 -> Divide3/1

== system Vessel/Time varying elastance1/k/Subsystem1 ==
  t : Inport
  "f(g1, g2)" : Inport  Port=2
  MinMax Running Resettable1 : simulink/Math Operations/MinMax Running Resettable  Function=max  vinit=0
      settings: AttributesFormatString=%<vinit>
  Pulse Generator1 : DiscretePulseGenerator  PulseType=Time based  TimeSource=Use external signal  Period=100  PulseWidth=1e-3
  Sample and Hold1 : dspsigops/Sample and Hold  trig=Rising edge  initCond=0.5  latchinput=on
  Saturation : Saturate  UpperLimit=inf  LowerLimit=0.5
  "max(f(g1, g2))" : Outport
  wires:
  "f(g1, g2)"/1 -> MinMax Running Resettable1/1
  MinMax Running Resettable1/1 -> Sample and Hold1/1
  t/1 -> Pulse Generator1/1
  Sample and Hold1/1 -> Saturation/1  "max(f(g1, g2))"
  Pulse Generator1/1 -> MinMax Running Resettable1/2, Sample and Hold1/Trigger
  Saturation/1 -> "max(f(g1, g2))"/1

== system Vessel/Total heart/Aortic Flow Target/Subsystem ==
  In1 : Inport
  IsNaN : RelationalOperator  Operator=isNaN  OutDataTypeStr=boolean  RndMeth=Simplest  InputSameDT=off
  IsZero : simulink/Logic and Bit Operations/Compare To Zero  relop===  OutDataTypeStr=boolean
      settings: LibrarySourceBlock=|
      | simulink/Quick Insert/Logic and Bit
      | Operations/IsZero
  NOT : Logic  Operator=NOT  IconShape=distinctive  AllPortsSameDT=off  OutDataTypeStr=boolean
  OR : Logic  Operator=OR  IconShape=distinctive  AllPortsSameDT=off  OutDataTypeStr=boolean
  Out1 : Outport
  wires:
  In1/1 -> IsNaN/1, IsZero/1
  NOT/1 -> Out1/1
  IsNaN/1 -> OR/1
  IsZero/1 -> OR/2
  OR/1 -> NOT/1

== system Vessel/Total heart/Heart beat/Subsystem ==
  t : Inport
  Constant1 : Constant
  Data Store Read2 : DataStoreRead  DataStoreName=T  IndexOptions=Index vector (dialog)  Indices=1  OutputSizes=1
  Gain : Gain  Gain=0.5
  Memory3 : Memory  InheritSampleTime=on
  Memory4 : Memory  InheritSampleTime=on
  Minus1 : Sum  Inputs=+-
  Minus4 : Sum
  Mod2 : Math  Operator=mod
  Product2 : Product
  Product3 : Product
  Reciprocal1 : Product  Inputs=/
  tag scope: t_b_2x=global
  wires:
  Memory3/1 -> Minus1/2
  Constant1/1 -> Mod2/2
  Mod2/1 -> Memory4/1, Product3/1
  Gain/1 -> Reciprocal1/1, Product3/2
  t/1 -> Memory3/1, Minus1/1
  Minus1/1 -> Product2/1
  Product3/1 -> [t_b_2x]
  Minus4/1 -> Mod2/1
  Product2/1 -> Minus4/2
  Reciprocal1/1 -> Product2/2
  Data Store Read2/1 -> Gain/1  "T"
  Memory4/1 -> Minus4/1

== system Vessel/Valve1/Subsystem/radius ==
  A_eff(t) : Inport
  Gain1 : Gain  Gain=1/pi
  Sqrt : Sqrt
  r(t) : Outport
  wires:
  Sqrt/1 -> r(t)/1
  A_eff(t)/1 -> Gain1/1
  Gain1/1 -> Sqrt/1

== matlab function Vessel/UVV Control/MATLAB Function ==
  data: u input
  events: trigger input FALLING_EDGE_EVENT
function fn(u)

coder.extrinsic('set_param')
set_param(['' bdroot '/UVV Control/K_uvv'],'Value',sprintf('%.2f',u));

== matlab function Vessel/SLVP control/MATLAB Function ==
  data: u input
  events: trigger input FALLING_EDGE_EVENT
function fn(u)

coder.extrinsic('set_param')
set_param(['' bdroot '/SLVP control/K_LV_Emax'],'Value',sprintf('%.2f',u));

== matlab function Vessel/Valve1/MATLAB Function ==
  data: A_eff input; xi input; B output; rho input; L output
function [B,L] = fcn(A_eff,xi, rho)

%Inputs
% B = Bernoulli resistance
% L = Inertance

r=sqrt(abs(A_eff/pi));
B = rho/(2*abs(A_eff)^2*(980.665*1.3595101283313));
L = rho*2/((pi*r)*980.665*1.3595101283313);

== matlab function Vessel/SRVP control/MATLAB Function ==
  data: u input
  events: trigger input FALLING_EDGE_EVENT
function fn(u)

coder.extrinsic('set_param')
set_param(['' bdroot '/SRVP control/K_RV_Emax'],'Value',sprintf('%.2f',u));

== matlab function Vessel/SAP//DAP control/MATLAB Function ==
  data: u input
  events: trigger input FALLING_EDGE_EVENT
function fn(u)

coder.extrinsic('set_param')
set_param(['' bdroot '/SAP//DAP control/K_Y_aorta'],'Value',sprintf('%.2f',u));

== matlab function Vessel/SPP//DPP control/MATLAB Function ==
  data: u input
  events: trigger input FALLING_EDGE_EVENT
function fn(u)

coder.extrinsic('set_param')
set_param(['' bdroot '/SPP//DPP control/K_Y_pulmonary_arteries'],'Value',sprintf('%.2f',u));

== matlab function Vessel/Time varying elastance (old)/MATLAB Function ==
  data: m1_ref input; E output; m2_ref input; alpha1_ref input; alpha2_ref input; E_max input; E_min input; t input; T input; sigma input; V_0 input; V input; V_max input; q input; Q_max input; v_ed input; e_min output; e_max output; t_delay input
function [E, e_min, e_max] = fcn(m1_ref, m2_ref, alpha1_ref, alpha2_ref, E_max, E_min, t, T, sigma, V_0, V, V_max, q, Q_max, v_ed, t_delay)

%Cardiac parameters correctiondue to varying cardiac cycle
m1 = m1_ref*T^0.5;
m2 = m2_ref/T^0.5;
alpha1 = alpha1_ref/T^0.7;
alpha2 = alpha2_ref/T^0.7;
tau1 = T*alpha1;
tau2 = T*alpha2;

%Maximum and minum elastances
e_min = E_min*exp(sigma*(V-V_0));%v_0 is the residual volume
e_max = E_max*(1-(v_ed/V_max)^4)*(1-q/Q_max);

% Define the function f(t)
f = @(t) (t/tau1)^m1 / (1 + (t/tau1)^m1) * 1 / (1 + (t/tau2)^m2);

% Set the time window to compute
t_start = 0;
t_end = T;

%Find the location of maximum
tmax = fminbnd(@(t) -f(t), t_start, t_end);
%tmax = T*025;
% tmax = T^2*(m2_ref*alpha1_ref^2-alpha2_ref)/(m1_ref)+ T*(alpha2_ref/(m2_ref)^(alpha1_ref/alpha2_ref))+alpha1_ref/(m1_ref^alpha2_ref);

%Calculate normalization factor
g1 = (tmax./tau1).^m1;
g2 = (tmax./tau2).^m2;
k = (e_max-e_min)/max((g1./(1+g1)).*(1./(1+g2)));% For dynamic elastance  (remember to comment this line)
%Calculate time Varying elastance
t2 = (t-t_delay)*((t-t_delay)>=0);
g1 = (t2./tau1).^m1;
g2 = (t2./tau2).^m2;
E = k*(g1/(1+g1))*(1/(1+g2))+e_min;       % For dynamic elastance  (remember to comment this line)

== matlab function Vessel/SVR Control/MATLAB Function ==
  data: u input
  events: trigger input FALLING_EDGE_EVENT
function fn(u)

coder.extrinsic('set_param')
set_param(['' bdroot '/SVR Control/K_svr'],'Value',sprintf('%.2f',u));

== matlab function Vessel/PVR Control/MATLAB Function ==
  data: u input
  events: trigger input FALLING_EDGE_EVENT
function fn(u)

coder.extrinsic('set_param')
set_param(['' bdroot '/PVR Control/K_pvr'],'Value',sprintf('%.2f',u));
